simulink library "mach_lib"  (Simulink 6.3)
undefined symbols (not defined in the file): accel_cmd, aero_surf_qbar_off, aero_surf_qbar_on, altitude_stop, angular_rate_stop, att_cmd_select, att_trim_IC, att_type, att_type_numbers, bb_ellipsoid, bb_params, chi_trim_IC, command_time, compute_all_rate_cols, compute_all_vel_cols, constants, cosA, da_trim_IC, de_trim_IC, DiscIntNeverNeededParam, dr_trim_IC, dtsim, E_rwy, E_trim_IC, Ed_cmd, Ed_trim_IC, energy_stop, eow_boundary, full_surf_llim, full_surf_ulim, gain_var_struct, gam_cmd_descent, gam_cmd_preflare, gamdot_cmd_descent, gamdot_cmd_flare, gamdot_cmd_preflare, gamma_trim_IC, h_trim_IC, hd_cmd, hd_trim_IC, ideal_vel_Kb, integrate_start_time_sim, integrate_state_sim, llim, MACH, MACH_att_fb, MACH_gain_mat, MACH_mass_IC, MACH_pos_IC, MACH_pqr_Bmat_IC, MACH_pqr_IC, MACH_pqr_u_IC, MACH_quat_IC, MACH_throttle_IC, MACH_U_nom_IC, MACH_vel_Bmat_IC, MACH_vel_cvdnom_IC, MACH_vel_IC, MACH_vel_uold_IC, max_chi_cmd ... (+67)
libraries: simulink x75, mach_lib x27, utility_lib x25, model_lib x7, models x6
(part 1 of 6)
settings Model: Creator=spratt  LastModifiedBy=E700252  ExtModeAutoUpdateStatusClock=off  StrictBusMsg=None

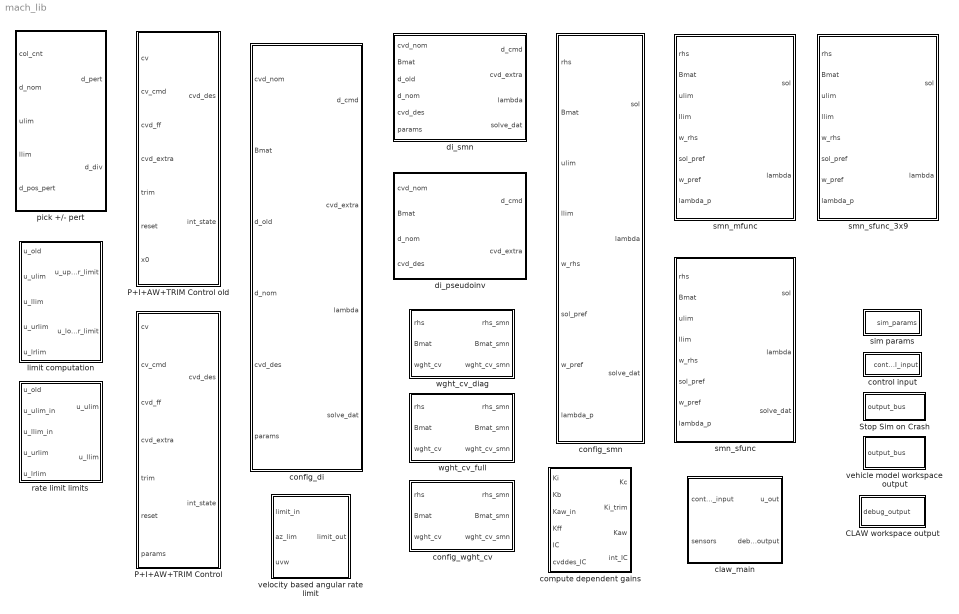
== system mach_lib ==
  CLAW workspace output : Subsystem
  P+I+AW+TRIM Control : Subsystem
  P+I+AW+TRIM Control old : Subsystem  mask{kb=MACH.xxx_Kb, ki=MACH.xxx_Ki, kc=MACH.xxx_Kc, kf=MACH.xxx_Kf, kaw=MACH.xxx_Kaw}
      mask prompts: kb "Kb (bandwidth gain)"; ki "Ki (integral gain)"; kc "Kc (command gain)"; kf "Kf (feedforward gain)"; kaw "Kaw (anti-windup gain)"
  Stop Sim on Crash : Subsystem
  claw_main : Subsystem  TreatAsAtomicUnit=on  SystemSampleTime=MACH.dt
  compute dependent gains : Subsystem
  config_di : Subsystem  BlockChoice=di_smn  mask{num_cv=0, num_u=0, wght_cv_type=0}
      settings: TemplateBlock=self  MemberBlocks=di_pseudoinv,di_smn
  config_smn : Subsystem  BlockChoice=smn_sfunc  mask{nr=num_cv, nc=num_u}
      settings: TemplateBlock=self  MemberBlocks=smn_mfunc,smn_sfunc,smn_sfunc_3x9
  config_wght_cv : Subsystem  BlockChoice=wght_cv_diag  mask{wght_cv_type=wght_cv_type}
      mask init:
      | try
      |     set_param(gcb, 'BlockChoice', wght_cv_type);
      | catch
      | %     disp(sprintf('resetting %s to default', gcb))
      | %     set_param(gcb, 'BlockChoice', 'wght_cv_diag');
      | end
      settings: TemplateBlock=self  MemberBlocks=wght_cv_diag,wght_cv_full
  control input : Subsystem  SystemSampleTime=MACH.dt
  di_pseudoinv : Subsystem
  di_smn : Subsystem
  limit computation : Subsystem
  pick +/- pert : Subsystem  mask{num_u=0}
  rate limit limits : Subsystem  mask{ulim=ulim, llim=llim}
      mask prompts: ulim "upper limit"; llim "lower limit"
  sim params : Subsystem
  smn_mfunc : Subsystem
  smn_sfunc : Subsystem  mask{sfunc_name=MACH.smn_sfunc_name}
      mask prompts: sfunc_name "S-function name"
      mask init:
      | block_name = [gcb '/S-Function'];
      | % disp(sprintf('S-Function name = %s',sfunc_name))
      | try
      |     set_param(block_name,'FunctionName',sfunc_name);
      | %     disp(sprintf('setting %s to %s',block_name,sfunc_name));
      | catch
      |     set_param(block_name,'FunctionName','smn_sfunc_3x9');
      | %     disp(sprintf('trouble setting smn_sfunc to %s, resetting %s to %s',sfunc_name,block_name,'smn_sfunc'));
      | end
  smn_sfunc_3x9 : Subsystem
  vehicle model workspace output : Subsystem
  velocity based angular rate limit : Subsystem  mask{q_idx=2}
      mask prompts: q_idx "q index"
  wght_cv_diag : Subsystem
  wght_cv_full : Subsystem

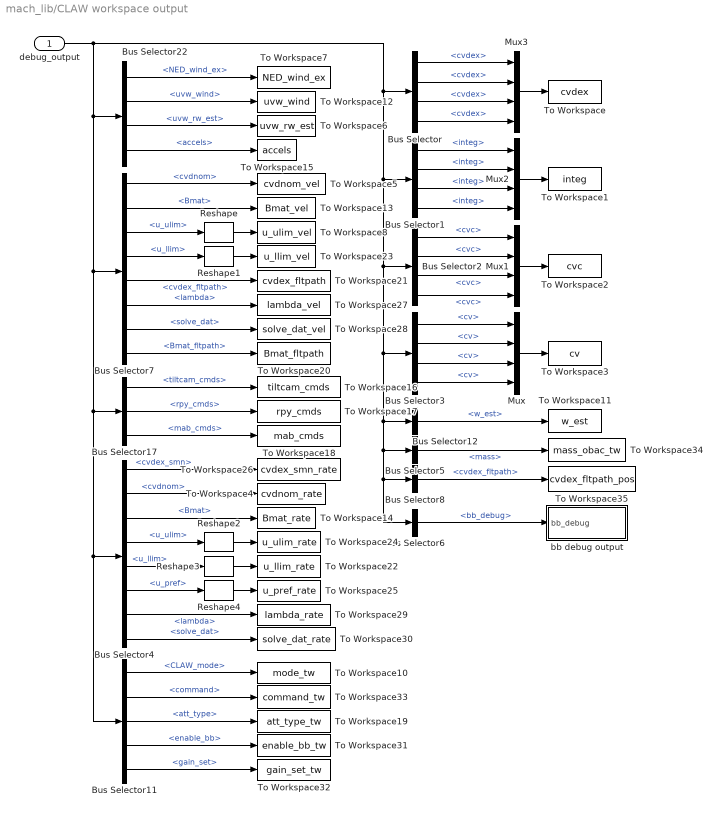
== system mach_lib/CLAW workspace output ==
  debug_output : Inport
  Bus Selector : BusSelector  OutputSignals=rate.cvdex,att.cvdex,vel.cvdex,pos.cvdex
  Bus Selector1 : BusSelector  OutputSignals=rate.integ,att.integ,vel.integ,pos.integ
  Bus Selector11 : BusSelector  OutputSignals=control_input.mode_sw.CLAW_mode,control_input.command,att_type,enable_bb,gain_set
  Bus Selector12 : BusSelector  OutputSignals=w_est_debug.w_est
  Bus Selector17 : BusSelector  OutputSignals=att.tiltcam_cmds,att.rpy_cmds,att.mab_cmds
  Bus Selector2 : BusSelector  OutputSignals=rate.cvc,att.cvc,vel.cvc,pos.cvc
  Bus Selector22 : BusSelector  OutputSignals=w_est_debug.NED_wind_ex,w_est_debug.uvw_wind,w_est_debug.uvw_rw_est,w_est_debug.accels
  Bus Selector3 : BusSelector  OutputSignals=rate.cv,att.cv,vel.cv,pos.cv
  Bus Selector4 : BusSelector  OutputSignals=rate.cvdex_smn,rate.cvdnom,rate.Bmat,rate.u_ulim,rate.u_llim,rate.u_pref,rate.lambda,rate.solve_dat
  Bus Selector5 : BusSelector  OutputSignals=mass
  Bus Selector6 : BusSelector  OutputSignals=rate.bb_debug
  Bus Selector7 : BusSelector  OutputSignals=vel.cvdnom,vel.Bmat,vel.u_ulim,vel.u_llim,vel.cvdex_fltpath,vel.lambda,vel.solve_dat,vel.Bmat_fltpath
  Bus Selector8 : BusSelector  OutputSignals=pos.cvdex_fltpath
  Mux{,1..3} (4 alike) : Mux
  Reshape{,1..4} (5 alike) : simulink/Math Operations/Reshape  OutputDimensionality=1-D array  OutputDimensions=[1,1]
  To Workspace : ToWorkspace  VariableName=cvdex  SampleTime=-1  SaveFormat=Array
  To Workspace1 : ToWorkspace  VariableName=integ  SampleTime=-1  SaveFormat=Array
  To Workspace10 : ToWorkspace  VariableName=mode_tw  SampleTime=-1  SaveFormat=Array
  To Workspace11 : ToWorkspace  VariableName=w_est  SampleTime=-1  SaveFormat=Array
  To Workspace12 : ToWorkspace  VariableName=uvw_wind  SampleTime=-1  SaveFormat=Array
  To Workspace13 : ToWorkspace  VariableName=Bmat_vel  SampleTime=-1  SaveFormat=Array
  To Workspace14 : ToWorkspace  VariableName=Bmat_rate  SampleTime=-1  SaveFormat=Array
  To Workspace15 : ToWorkspace  VariableName=accels  SampleTime=-1  SaveFormat=Array
  To Workspace16 : ToWorkspace  VariableName=tiltcam_cmds  SampleTime=-1  SaveFormat=Array
  To Workspace17 : ToWorkspace  VariableName=rpy_cmds  SampleTime=-1  SaveFormat=Array
  To Workspace18 : ToWorkspace  VariableName=mab_cmds  SampleTime=-1  SaveFormat=Array
  To Workspace19 : ToWorkspace  VariableName=att_type_tw  SampleTime=-1  SaveFormat=Array
  To Workspace2 : ToWorkspace  VariableName=cvc  SampleTime=-1  SaveFormat=Array
  To Workspace20 : ToWorkspace  VariableName=Bmat_fltpath  SampleTime=-1  SaveFormat=Array
  To Workspace21 : ToWorkspace  VariableName=cvdex_fltpath  SampleTime=-1  SaveFormat=Array
  To Workspace22 : ToWorkspace  VariableName=u_llim_rate  SampleTime=-1  SaveFormat=Array
  To Workspace23 : ToWorkspace  VariableName=u_llim_vel  SampleTime=-1  SaveFormat=Array
  To Workspace24 : ToWorkspace  VariableName=u_ulim_rate  SampleTime=-1  SaveFormat=Array
  To Workspace25 : ToWorkspace  VariableName=u_pref_rate  SampleTime=-1  SaveFormat=Array
  To Workspace26 : ToWorkspace  VariableName=cvdex_smn_rate  SampleTime=-1  SaveFormat=Array
  To Workspace27 : ToWorkspace  VariableName=lambda_vel  SampleTime=-1  SaveFormat=Array
  To Workspace28 : ToWorkspace  VariableName=solve_dat_vel  SampleTime=-1  SaveFormat=Array
  To Workspace29 : ToWorkspace  VariableName=lambda_rate  SampleTime=-1  SaveFormat=Array
  To Workspace3 : ToWorkspace  VariableName=cv  SampleTime=-1  SaveFormat=Array
  To Workspace30 : ToWorkspace  VariableName=solve_dat_rate  SampleTime=-1  SaveFormat=Array
  To Workspace31 : ToWorkspace  VariableName=enable_bb_tw  SampleTime=-1  SaveFormat=Array
  To Workspace32 : ToWorkspace  VariableName=gain_set_tw  SampleTime=-1  SaveFormat=Array
  To Workspace33 : ToWorkspace  VariableName=command_tw  SampleTime=-1  SaveFormat=Array
  To Workspace34 : ToWorkspace  VariableName=mass_obac_tw  SampleTime=-1  SaveFormat=Array
  To Workspace35 : ToWorkspace  VariableName=cvdex_fltpath_pos  SampleTime=-1  SaveFormat=Array
  To Workspace4 : ToWorkspace  VariableName=cvdnom_rate  SampleTime=-1  SaveFormat=Array
  To Workspace5 : ToWorkspace  VariableName=cvdnom_vel  SampleTime=-1  SaveFormat=Array
  To Workspace6 : ToWorkspace  VariableName=uvw_rw_est  SampleTime=-1  SaveFormat=Array
  To Workspace7 : ToWorkspace  VariableName=NED_wind_ex  SampleTime=-1  SaveFormat=Array
  To Workspace8 : ToWorkspace  VariableName=u_ulim_vel  SampleTime=-1  SaveFormat=Array
  bb debug output : Subsystem
  wires:
  Bus Selector8/1 -> To Workspace35/1  "<cvdex_fltpath>"
  Bus Selector6/1 -> bb debug output/1(bb_debug)  "<bb_debug>"
  Bus Selector5/1 -> To Workspace34/1  "<mass>"
  Bus Selector11/5 -> To Workspace32/1  "<gain_set>"
  Bus Selector11/4 -> To Workspace31/1  "<enable_bb>"
  Bus Selector7/8 -> To Workspace20/1  "<Bmat_fltpath>"
  Bus Selector4/8 -> To Workspace30/1  "<solve_dat>"
  Bus Selector4/7 -> To Workspace29/1  "<lambda>"
  Bus Selector7/7 -> To Workspace28/1  "<solve_dat>"
  Bus Selector7/6 -> To Workspace27/1  "<lambda>"
  Bus Selector4/1 -> To Workspace26/1  "<cvdex_smn>"
  Reshape4/1 -> To Workspace25/1
  Bus Selector4/6 -> Reshape4/1  "<u_pref>"
  Reshape3/1 -> To Workspace22/1
  Reshape2/1 -> To Workspace24/1
  Reshape1/1 -> To Workspace23/1
  Reshape/1 -> To Workspace8/1
  Bus Selector4/5 -> Reshape3/1  "<u_llim>"
  Bus Selector4/4 -> Reshape2/1  "<u_ulim>"
  Bus Selector4/3 -> To Workspace14/1  "<Bmat>"
  Bus Selector4/2 -> To Workspace4/1  "<cvdnom>"
  Bus Selector7/5 -> To Workspace21/1  "<cvdex_fltpath>"
  Bus Selector7/4 -> Reshape1/1  "<u_llim>"
  Bus Selector7/3 -> Reshape/1  "<u_ulim>"
  Bus Selector7/2 -> To Workspace13/1  "<Bmat>"
  Bus Selector7/1 -> To Workspace5/1  "<cvdnom>"
  Bus Selector22/4 -> To Workspace15/1  "<accels>"
  Bus Selector22/3 -> To Workspace6/1  "<uvw_rw_est>"
  Bus Selector22/2 -> To Workspace12/1  "<uvw_wind>"
  Bus Selector22/1 -> To Workspace7/1  "<NED_wind_ex>"
  Bus Selector11/2 -> To Workspace33/1  "<command>"
  Bus Selector11/1 -> To Workspace10/1  "<CLAW_mode>"
  Bus Selector17/3 -> To Workspace18/1  "<mab_cmds>"
  Bus Selector17/2 -> To Workspace17/1  "<rpy_cmds>"
  Bus Selector17/1 -> To Workspace16/1  "<tiltcam_cmds>"
  Bus Selector12/1 -> To Workspace11/1  "<w_est>"
  Bus Selector11/3 -> To Workspace19/1  "<att_type>"
  debug_output/1 -> Bus Selector4/1, Bus Selector11/1, Bus Selector17/1, Bus Selector7/1, Bus Selector22/1, Bus Selector8/1, Bus Selector6/1, Bus Selector5/1, Bus Selector12/1, Bus Selector3/1, Bus Selector2/1, Bus Selector1/1, Bus Selector/1
  Bus Selector3/1 -> Mux/1  "<cv>"
  Bus Selector3/2 -> Mux/2  "<cv>"
  Bus Selector3/3 -> Mux/3  "<cv>"
  Bus Selector3/4 -> Mux/4  "<cv>"
  Mux/1 -> To Workspace3/1
  Bus Selector2/1 -> Mux1/1  "<cvc>"
  Bus Selector2/2 -> Mux1/2  "<cvc>"
  Bus Selector2/3 -> Mux1/3  "<cvc>"
  Bus Selector2/4 -> Mux1/4  "<cvc>"
  Mux1/1 -> To Workspace2/1
  Bus Selector1/1 -> Mux2/1  "<integ>"
  Bus Selector1/2 -> Mux2/2  "<integ>"
  Bus Selector1/3 -> Mux2/3  "<integ>"
  Bus Selector1/4 -> Mux2/4  "<integ>"
  Mux2/1 -> To Workspace1/1
  Bus Selector/1 -> Mux3/1  "<cvdex>"
  Bus Selector/2 -> Mux3/2  "<cvdex>"
  Bus Selector/3 -> Mux3/3  "<cvdex>"
  Bus Selector/4 -> Mux3/4  "<cvdex>"
  Mux3/1 -> To Workspace/1

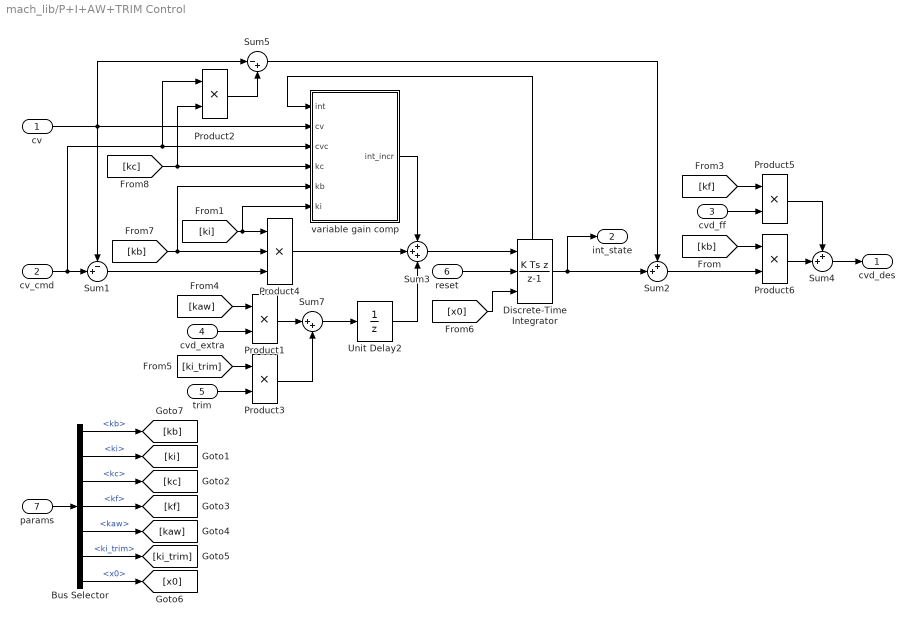
== system mach_lib/P+I+AW+TRIM Control ==
  cv : Inport
  cv_cmd : Inport  Port=2
  cvd_ff : Inport  Port=3
  cvd_extra : Inport  Port=4
  trim : Inport  Port=5
  reset : Inport  Port=6
  params : Inport  Port=7
  Bus Selector : BusSelector  OutputSignals=kb,ki,kc,kf,kaw,ki_trim,x0
  Discrete-Time Integrator : DiscreteIntegrator  IntegratorMethod=Integration: Backward Euler  ExternalReset=rising  InitialConditionSource=external  SampleTime=-1  ShowStatePort=on  ICPrevOutput=DiscIntNeverNeededParam  ICPrevScaledInput=DiscIntNeverNeededParam
  Product{1..3,5..6} (5 alike) : Product  RndMeth=Zero
  Product4 : Product  Inputs=3  RndMeth=Zero
  Sum1 : Sum  Inputs=-+|  SaturateOnIntegerOverflow=on  InputSameDT=on
  Sum2 : Sum  Inputs=++|  SaturateOnIntegerOverflow=on  InputSameDT=on
  Sum3 : Sum  Inputs=+++  SaturateOnIntegerOverflow=on  InputSameDT=on
  Sum4 : Sum  Inputs=++|  SaturateOnIntegerOverflow=on  InputSameDT=on
  Sum5 : Sum  Inputs=|-+  SaturateOnIntegerOverflow=on  InputSameDT=on
  Sum7 : Sum  Inputs=|++  SaturateOnIntegerOverflow=on  InputSameDT=on
  Unit Delay2 : UnitDelay  SampleTime=-1
  variable gain comp : Subsystem
  cvd_des : Outport
  int_state : Outport  Port=2
  wires:
  [x0] -> Discrete-Time Integrator/3
  Product5/1 -> Sum4/1
  Sum4/1 -> cvd_des/1
  Product6/1 -> Sum4/2
  trim/1 -> Product3/2
  Unit Delay2/1 -> Sum3/3
  Sum3/1 -> Discrete-Time Integrator/1
  Discrete-Time Integrator/1 -> int_state/1, Sum2/2
  cvd_extra/1 -> Product1/2
  reset/1 -> Discrete-Time Integrator/2
  Product3/1 -> Sum7/2
  Sum7/1 -> Unit Delay2/1
  Bus Selector/1 -> [kb]  "<kb>"
  Bus Selector/2 -> [ki]  "<ki>"
  Bus Selector/3 -> [kc]  "<kc>"
  Bus Selector/4 -> [kf]  "<kf>"
  Bus Selector/5 -> [kaw]  "<kaw>"
  Bus Selector/6 -> [ki_trim]  "<ki_trim>"
  [kaw] -> Product1/1
  Product1/1 -> Sum7/1
  [ki_trim] -> Product3/1
  Sum1/1 -> Product4/3
  [ki] -> Product4/1, variable gain comp/6(ki)
  [kb] -> Product6/1
  cvd_ff/1 -> Product5/2
  [kf] -> Product5/1
  params/1 -> Bus Selector/1
  Bus Selector/7 -> [x0]  "<x0>"
  cv/1 -> Sum1/1, Sum5/1, variable gain comp/2(cv)
  Sum2/1 -> Product6/2
  Product4/1 -> Sum3/2
  variable gain comp/1(int_incr) -> Sum3/1
  Discrete-Time Integrator/State -> variable gain comp/1(int)
  [kc] -> variable gain comp/4(kc), Product2/2
  Product2/1 -> Sum5/2
  Sum5/1 -> Sum2/1
  [kb] -> Product4/2, variable gain comp/5(kb)
  cv_cmd/1 -> variable gain comp/3(cvc), Product2/1, Sum1/2

== system mach_lib/P+I+AW+TRIM Control old ==
  cv : Inport
  cv_cmd : Inport  Port=2
  cvd_ff : Inport  Port=3
  cvd_extra : Inport  Port=4
  trim : Inport  Port=5
  reset : Inport  Port=6
  x0 : Inport  Port=7
  Discrete-Time Integrator : DiscreteIntegrator  IntegratorMethod=Integration: Backward Euler  ExternalReset=rising  InitialConditionSource=external  SampleTime=-1  ICPrevOutput=DiscIntNeverNeededParam  ICPrevScaledInput=DiscIntNeverNeededParam
  Kaw : Gain  Gain=kaw  SaturateOnIntegerOverflow=on
  Kb : Gain  Gain=kb  SaturateOnIntegerOverflow=on
  Kb1 : Gain  Gain=kb  SaturateOnIntegerOverflow=on
  Kc : Gain  Gain=kc  SaturateOnIntegerOverflow=on
  Kf : Gain  Gain=kf  SaturateOnIntegerOverflow=on
  Ki : Gain  Gain=ki  SaturateOnIntegerOverflow=on
  Sum1 : Sum  Inputs=|+-  SaturateOnIntegerOverflow=on  InputSameDT=on
  Sum2 : Sum  Inputs=|++  SaturateOnIntegerOverflow=on  InputSameDT=on
  Sum3 : Sum  Inputs=|++  SaturateOnIntegerOverflow=on  InputSameDT=on
  Sum4 : Sum  Inputs=++|  SaturateOnIntegerOverflow=on  InputSameDT=on
  Sum5 : Sum  Orientation=up  Inputs=++|  SaturateOnIntegerOverflow=on
  Sum6 : Sum  Inputs=-+|  SaturateOnIntegerOverflow=on  InputSameDT=on
  Unit Delay1 : UnitDelay  SampleTime=-1
  cvd_des : Outport
  int_state : Outport  Port=2
  wires:
  reset/1 -> Discrete-Time Integrator/2
  cvd_extra/1 -> Unit Delay1/1
  Discrete-Time Integrator/1 -> int_state/1, Sum2/1
  Sum3/1 -> Discrete-Time Integrator/1
  Ki/1 -> Sum3/1
  cv_cmd/1 -> Sum1/1, Kc/1
  Sum2/1 -> Kb/1
  cv/1 -> Sum1/2, Sum6/1
  Sum1/1 -> Kb1/1
  Kb1/1 -> Ki/1
  Sum5/1 -> Sum3/2
  Kaw/1 -> Sum5/1
  trim/1 -> Sum5/2
  Unit Delay1/1 -> Kaw/1
  Kb/1 -> Sum4/2
  Sum4/1 -> cvd_des/1
  cvd_ff/1 -> Kf/1
  Kf/1 -> Sum4/1
  Kc/1 -> Sum6/2
  Sum6/1 -> Sum2/2
  x0/1 -> Discrete-Time Integrator/3

== system mach_lib/Stop Sim on Crash ==
  note: If angular rates exceed 2 rad/sec, stop simulation
      |  because vehicle most likely crashed
  output_bus : Inport
  Abs : Abs  SaturateOnIntegerOverflow=on
  Bus Selector2 : BusSelector  OutputSignals=x,xdot
  Constant1 : Constant  Value=angular_rate_stop
  Constant2 : Constant  Value=altitude_stop
  Constant3 : Constant  Value=energy_stop
  MinMax : MinMax  Function=max  SaturateOnIntegerOverflow=on  InputSameDT=on
  NEh_dot : Selector  Elements=MACH.NEh_idx  InputPortWidth=trac_params.num_x
  Relational Operator1 : RelationalOperator  Operator=>
  Relational Operator2 : RelationalOperator  Operator=<
  Relational Operator3 : RelationalOperator  Operator=<
  Stop Simulation : Stop
  Stop Simulation1 : Stop
  Stop Simulation2 : Stop
  get specific energy : Subsystem
  h : Selector  Elements=MACH.NEh_idx(3)  InputPortWidth=MACH.num_x
  pqr : Selector  Elements=MACH.pqr_idx  InputPortWidth=trac_params.num_x
  wires:
  Abs/1 -> MinMax/1
  MinMax/1 -> Relational Operator1/1
  Relational Operator1/1 -> Stop Simulation/1
  Constant1/1 -> Relational Operator1/2
  pqr/1 -> Abs/1
  output_bus/1 -> Bus Selector2/1
  Constant2/1 -> Relational Operator2/2
  h/1 -> get specific energy/1(h), Relational Operator2/1
  Relational Operator2/1 -> Stop Simulation1/1
  Constant3/1 -> Relational Operator3/2
  get specific energy/1(energy) -> Relational Operator3/1
  Relational Operator3/1 -> Stop Simulation2/1
  Bus Selector2/1 -> h/1, pqr/1  "<x>"
  NEh_dot/1 -> get specific energy/2(NEh_dot)
  Bus Selector2/2 -> NEh_dot/1  "<xdot>"

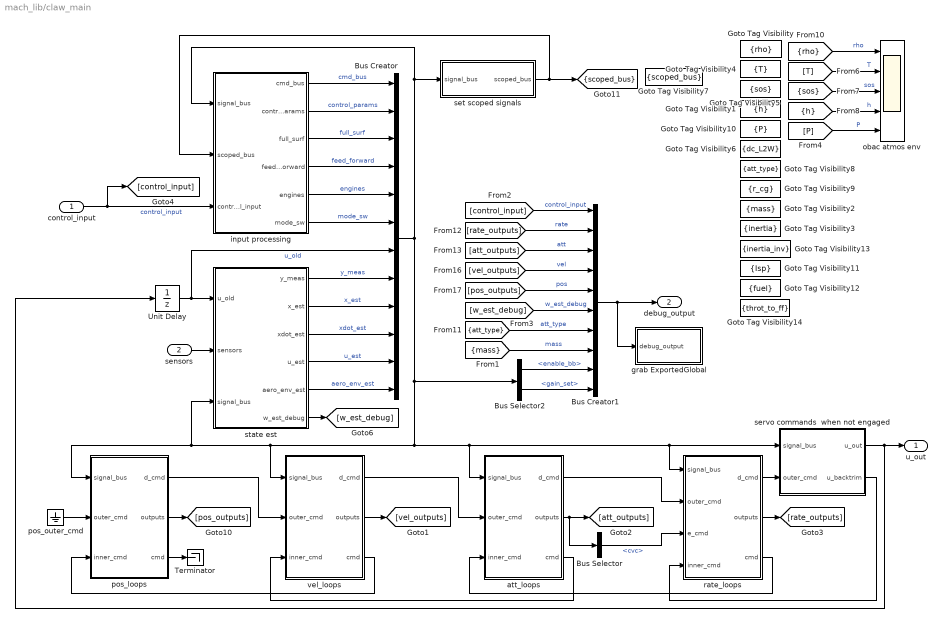
== system mach_lib/claw_main ==
  control_input : Inport
      settings: BusObject=control_input_bus
  sensors : Inport  Port=2
  Bus Creator : BusCreator  Inputs=12
  Bus Creator1 : BusCreator  Inputs=10
      settings: BusObject=CLAW_DEBUG_OUTPUT_BUS
  Bus Selector : BusSelector  OutputSignals=cvc
  Bus Selector2 : BusSelector  OutputSignals=control_params.enable_bb,control_params.gain_set
  Goto Tag Visibility : GotoTagVisibility  GotoTag=rho
  Goto Tag Visibility1 : GotoTagVisibility  GotoTag=h
  Goto Tag Visibility10 : GotoTagVisibility  GotoTag=P
  Goto Tag Visibility11 : GotoTagVisibility  GotoTag=Isp
  Goto Tag Visibility12 : GotoTagVisibility  GotoTag=fuel
  Goto Tag Visibility13 : GotoTagVisibility  GotoTag=inertia_inv
  Goto Tag Visibility14 : GotoTagVisibility  GotoTag=throt_to_ff
  Goto Tag Visibility2 : GotoTagVisibility  GotoTag=mass
  Goto Tag Visibility3 : GotoTagVisibility  GotoTag=inertia
  Goto Tag Visibility4 : GotoTagVisibility  GotoTag=T
  Goto Tag Visibility5 : GotoTagVisibility  GotoTag=sos
  Goto Tag Visibility6 : GotoTagVisibility  GotoTag=dc_L2W
  Goto Tag Visibility7 : GotoTagVisibility  GotoTag=scoped_bus
  Goto Tag Visibility8 : GotoTagVisibility  GotoTag=att_type
  Goto Tag Visibility9 : GotoTagVisibility  GotoTag=r_cg
  Terminator : Terminator
  Unit Delay : UnitDelay  X0=MACH_U_nom_IC  SampleTime=-1
  att_loops : Subsystem
  grab ExportedGlobal : Subsystem
  input processing : Subsystem
  obac atmos env : Scope  NumInputPorts=5
      settings: YMin=-5~-5~-5~-5~-5  YMax=5~5~5~5~5  SaveName=ScopeData2
  pos_loops : Subsystem
      settings: RTWSystemCode=Function
  pos_outer_cmd : Ground
  rate_loops : Subsystem
      settings: RTWSystemCode=Function
  servo commands  when not engaged : Subsystem
  set scoped signals : Subsystem
  state est : Subsystem
  vel_loops : Subsystem
      settings: RTWSystemCode=Function
  u_out : Outport
  debug_output : Outport  Port=2
  tag scope: scoped_bus=scoped
  wires:
  Bus Selector/1 -> rate_loops/3(e_cmd)  "<cvc>"
  [control_input] -> Bus Creator1/1  "control_input"
  input processing/1(cmd_bus) -> Bus Creator/1  "cmd_bus"
  control_input/1 -> [control_input], input processing/3(control_input)  "control_input"
  Bus Selector2/2 -> Bus Creator1/10  "<gain_set>"
  Bus Selector2/1 -> Bus Creator1/9  "<enable_bb>"
  [mass] -> Bus Creator1/8  "mass"
  set scoped signals/1(scoped_bus) -> input processing/2(scoped_bus), [scoped_bus]
  input processing/4(feed_forward) -> Bus Creator/4  "feed_forward"
  input processing/3(full_surf) -> Bus Creator/3  "full_surf"
  state est/5(aero_env_est) -> Bus Creator/12  "aero_env_est"
  [P] -> obac atmos env/5  "P"
  [rho] -> obac atmos env/1  "rho"
  [T] -> obac atmos env/2  "T"
  [sos] -> obac atmos env/3  "sos"
  [h] -> obac atmos env/4  "h"
  input processing/2(control_params) -> Bus Creator/2  "control_params"
  [att_type] -> Bus Creator1/7  "att_type"
  [w_est_debug] -> Bus Creator1/6  "w_est_debug"
  state est/6(w_est_debug) -> [w_est_debug]
  pos_outer_cmd/1 -> pos_loops/2(outer_cmd)
  servo commands  when not engaged/1(u_out) -> Unit Delay/1, u_out/1
  state est/1(y_meas) -> Bus Creator/8  "y_meas"
  state est/2(x_est) -> Bus Creator/9  "x_est"
  state est/3(xdot_est) -> Bus Creator/10  "xdot_est"
  state est/4(u_est) -> Bus Creator/11  "u_est"
  servo commands  when not engaged/2(u_backtrim) -> rate_loops/4(inner_cmd)
  vel_loops/3(cmd) -> pos_loops/3(inner_cmd)
  sensors/1 -> state est/2(sensors)
  Unit Delay/1 -> Bus Creator/7, state est/1(u_old)  "u_old"
  Bus Creator1/1 -> grab ExportedGlobal/1(debug_output), debug_output/1
  rate_loops/2(outputs) -> [rate_outputs]
  att_loops/2(outputs) -> Bus Selector/1, [att_outputs]
  vel_loops/2(outputs) -> [vel_outputs]
  pos_loops/1(d_cmd) -> vel_loops/2(outer_cmd)
  rate_loops/3(cmd) -> att_loops/3(inner_cmd)
  att_loops/3(cmd) -> vel_loops/3(inner_cmd)
  pos_loops/3(cmd) -> Terminator/1
  Bus Creator/1 -> set scoped signals/1(signal_bus), input processing/1(signal_bus), Bus Selector2/1, state est/3(signal_bus), pos_loops/1(signal_bus), vel_loops/1(signal_bus), servo commands  when not engaged/1(signal_bus), rate_loops/1(signal_bus), att_loops/1(signal_bus)
  rate_loops/1(d_cmd) -> servo commands  when not engaged/2(outer_cmd)
  vel_loops/1(d_cmd) -> att_loops/2(outer_cmd)
  att_loops/1(d_cmd) -> rate_loops/2(outer_cmd)
  [rate_outputs] -> Bus Creator1/2  "rate"
  [att_outputs] -> Bus Creator1/3  "att"
  [vel_outputs] -> Bus Creator1/4  "vel"
  [pos_outputs] -> Bus Creator1/5  "pos"
  pos_loops/2(outputs) -> [pos_outputs]
  input processing/5(engines) -> Bus Creator/5  "engines"
  input processing/6(mode_sw) -> Bus Creator/6  "mode_sw"

== system mach_lib/compute dependent gains ==
  Ki : Inport
  Kb : Inport  Port=2
  Kaw_in : Inport  Port=3
  Kff : Inport  Port=4
  IC : Inport  Port=5
  cvddes_IC : Inport  Port=6
  Compare To Zero : simulink/Logic and Bit Operations/Compare To Zero  relop=>  LogicOutDataTypeMode=boolean  ZeroCross=off
  Constant : Constant
  Constant1 : Constant  Value=MACH.trim_loop_gain
  Constant2 : Constant
  Constant3 : Constant
  Constant4 : Constant  Value=0
  Divide : Product  Inputs=//**  OutScaling=2^-10
  Divide1 : Product  Inputs=**  OutScaling=2^-10
  Divide2 : Product  Inputs=**  OutScaling=2^-10
  Divide3 : Product  Inputs=/*  OutScaling=2^-10
  Gain : Gain  Gain=4
  Gain1 : Gain  Gain=0.5
  Math Function : Math  Operator=sqrt  SaturateOnIntegerOverflow=on
  Math Function1 : Math  Operator=sqrt  SaturateOnIntegerOverflow=on
  Sum : Sum  Inputs=|-+
  Sum1 : Sum  Inputs=|++
  Sum2 : Sum  Inputs=-+|
  Sum3 : Sum  Inputs=|++
  Switch : Switch  Threshold=0.25
  Switch1 : Switch  Threshold=1
  Switch2 : Switch  Threshold=1
  Kc : Outport
  Ki_trim : Outport  Port=2
  Kaw : Outport  Port=3
  int_IC : Outport  Port=4
  wires:
  Sum1/1 -> Gain1/1
  Math Function1/1 -> Sum1/1
  Sum/1 -> Math Function1/1
  Constant/1 -> Sum1/2, Sum/2
  Gain/1 -> Sum/1
  Math Function/1 -> Switch/1
  Gain1/1 -> Switch/3
  Ki/1 -> Switch/2, Math Function/1, Gain/1, Compare To Zero/1
  Switch/1 -> Switch1/3, Divide/2
  Constant1/1 -> Divide/3
  Divide/1 -> Ki_trim/1
  Compare To Zero/1 -> Divide/4, Divide1/1
  Kaw_in/1 -> Divide1/2
  Divide1/1 -> Kaw/1
  Constant2/1 -> Sum2/2
  Sum2/1 -> Divide2/1
  IC/1 -> Divide2/2
  Constant3/1 -> Switch1/1
  Kff/1 -> Switch1/2, Switch2/2
  Switch1/1 -> Sum2/1, Kc/1
  Divide3/1 -> Sum3/2
  Divide2/1 -> Sum3/1
  cvddes_IC/1 -> Divide3/2
  Kb/1 -> Divide/1, Divide3/1
  Constant4/1 -> Switch2/1
  Switch2/1 -> int_IC/1
  Sum3/1 -> Switch2/3

== system mach_lib/config_di ==
  cvd_nom : Inport
  Bmat : Inport  Port=2
  d_old : Inport  Port=3
  d_nom : Inport  Port=4
  cvd_des : Inport  Port=5
  params : Inport  Port=6
  di_smn : mach_lib/di_smn
  d_cmd : Outport
  cvd_extra : Outport  Port=2
  lambda : Outport  Port=3
  solve_dat : Outport  Port=4
  wires:
  cvd_nom/1 -> di_smn/1
  Bmat/1 -> di_smn/2
  d_old/1 -> di_smn/3
  d_nom/1 -> di_smn/4
  cvd_des/1 -> di_smn/5
  params/1 -> di_smn/6
  di_smn/1 -> d_cmd/1
  di_smn/2 -> cvd_extra/1
  di_smn/3 -> lambda/1
  di_smn/4 -> solve_dat/1

== system mach_lib/config_smn ==
  rhs : Inport
  Bmat : Inport  Port=2
  ulim : Inport  Port=3
  llim : Inport  Port=4
  w_rhs : Inport  Port=5
  sol_pref : Inport  Port=6
  w_pref : Inport  Port=7
  lambda_p : Inport  Port=8
  smn_sfunc : mach_lib/smn_sfunc  sfunc_name=smn_sfunc_name
  sol : Outport
  lambda : Outport  Port=2
  solve_dat : Outport  Port=3
  wires:
  rhs/1 -> smn_sfunc/1
  Bmat/1 -> smn_sfunc/2
  ulim/1 -> smn_sfunc/3
  llim/1 -> smn_sfunc/4
  w_rhs/1 -> smn_sfunc/5
  sol_pref/1 -> smn_sfunc/6
  w_pref/1 -> smn_sfunc/7
  lambda_p/1 -> smn_sfunc/8
  smn_sfunc/1 -> sol/1
  smn_sfunc/2 -> lambda/1
  smn_sfunc/3 -> solve_dat/1

== system mach_lib/config_wght_cv ==
  rhs : Inport
  Bmat : Inport  Port=2
  wght_cv : Inport  Port=3
  wght_cv_diag : mach_lib/wght_cv_diag
  rhs_smn : Outport
  Bmat_smn : Outport  Port=2
  wght_cv_smn : Outport  Port=3
  wires:
  rhs/1 -> wght_cv_diag/1
  Bmat/1 -> wght_cv_diag/2
  wght_cv/1 -> wght_cv_diag/3
  wght_cv_diag/1 -> rhs_smn/1
  wght_cv_diag/2 -> Bmat_smn/1
  wght_cv_diag/3 -> wght_cv_smn/1

== system mach_lib/control input ==
  Rate Transition1 : RateTransition  OutPortSampleTime=MACH.dt
  form control input : Subsystem  SystemSampleTime=MACH.dt
  generate commands : Subsystem
  ideal responses : model_lib/ideal responses
  control_input : Outport
  wires:
  generate commands/1(cmd_bus) -> form control input/1(cmd_bus)
  form control input/1(control_input) -> Rate Transition1/1
  Rate Transition1/1 -> control_input/1, ideal responses/1

== system mach_lib/di_pseudoinv ==
  cvd_nom : Inport
  Bmat : Inport  Port=2
  d_nom : Inport  Port=3
  cvd_des : Inport  Port=4
  Product : Product  Multiplication=Matrix(*)  SaturateOnIntegerOverflow=on  InputSameDT=on
  Sum : Sum  Inputs=|+-  SaturateOnIntegerOverflow=on  InputSameDT=on
  Sum4 : Sum  Inputs=|++  SaturateOnIntegerOverflow=on  InputSameDT=on
  Sum5 : Sum  Inputs=+-|  SaturateOnIntegerOverflow=on  InputSameDT=on
  pseudoinv : Subsystem
  d_cmd : Outport
  cvd_extra : Outport  Port=2
  wires:
  Product/1 -> Sum5/1
  cvd_des/1 -> Sum/1
  cvd_nom/1 -> Sum/2
  Bmat/1 -> pseudoinv/2(Bmat), Product/1
  Sum/1 -> pseudoinv/1(rhs), Sum5/2
  pseudoinv/1(sol) -> Sum4/1, Product/2
  d_nom/1 -> Sum4/2
  Sum4/1 -> d_cmd/1
  Sum5/1 -> cvd_extra/1

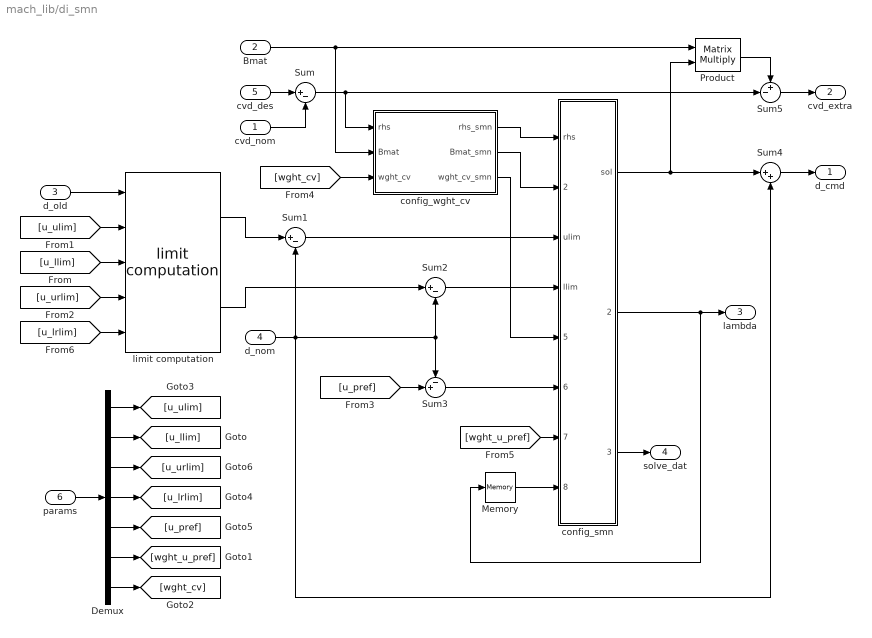
== system mach_lib/di_smn ==
  cvd_nom : Inport
  Bmat : Inport  Port=2
  d_old : Inport  Port=3
  d_nom : Inport  Port=4
  cvd_des : Inport  Port=5
  params : Inport  Port=6
  Demux : Demux  Outputs=7  BusSelectionMode=on
  Memory : Memory  InheritSampleTime=on
  Product : Product  Multiplication=Matrix(*)  SaturateOnIntegerOverflow=on  InputSameDT=on
  Sum : Sum  Inputs=|+-  SaturateOnIntegerOverflow=on  InputSameDT=on
  Sum1 : Sum  Inputs=|+-  SaturateOnIntegerOverflow=on  InputSameDT=on
  Sum2 : Sum  Inputs=|+-  SaturateOnIntegerOverflow=on  InputSameDT=on
  Sum3 : Sum  Inputs=-+|  SaturateOnIntegerOverflow=on  InputSameDT=on
  Sum4 : Sum  Inputs=|++  SaturateOnIntegerOverflow=on  InputSameDT=on
  Sum5 : Sum  Inputs=+-|  SaturateOnIntegerOverflow=on  InputSameDT=on
  config_smn : Subsystem  BlockChoice=smn_sfunc  mask{nr=num_cv, nc=num_u}
      link override smn_mfile: nr=num_cv  nc=num_u
      link override smn_sfunc: nr=num_cv  nc=num_u
      settings: AttributesFormatString=%<BlockChoice>  TemplateBlock=mach_lib/config_smn  MemberBlocks=smn_mfunc,smn_sfunc,smn_sfunc_3x9,smn_sfunc_old
  config_wght_cv : Subsystem  BlockChoice=wght_cv_diag  mask{wght_cv_type=wght_cv_type}
      mask init:
      | try
      |     set_param(gcb, 'BlockChoice', wght_cv_type);
      | catch
      |     disp(sprintf('resetting %s to default', gcb))
      |     set_param(gcb, 'BlockChoice', 'wght_cv_diag');
      | end
      settings: AttributesFormatString=%<BlockChoice>  TemplateBlock=mach_lib/config_wght_cv  MemberBlocks=wght_cv_diag,wght_cv_full
  limit computation : mach_lib/limit computation
  d_cmd : Outport
  cvd_extra : Outport  Port=2
  lambda : Outport  Port=3
  solve_dat : Outport  Port=4
  wires:
  [u_ulim] -> limit computation/2
  [u_llim] -> limit computation/3
  [u_urlim] -> limit computation/4
  d_old/1 -> limit computation/1
  Demux/7 -> [wght_cv]
  Demux/6 -> [wght_u_pref]
  Demux/5 -> [u_pref]
  Demux/4 -> [u_lrlim]
  Demux/2 -> [u_llim]
  Demux/1 -> [u_ulim]
  params/1 -> Demux/1
  [wght_u_pref] -> config_smn/7(w_pref)
  config_wght_cv/3(wght_cv_smn) -> config_smn/5(w_rhs)
  [u_pref] -> Sum3/2
  Product/1 -> Sum5/1
  cvd_des/1 -> Sum/1
  cvd_nom/1 -> Sum/2
  Bmat/1 -> Product/1, config_wght_cv/2(Bmat)
  Sum/1 -> Sum5/2, config_wght_cv/1(rhs)
  config_smn/1(sol) -> Sum4/1, Product/2
  limit computation/1 -> Sum1/1
  limit computation/2 -> Sum2/1
  d_nom/1 -> Sum4/2, Sum3/1, Sum2/2, Sum1/2
  Sum3/1 -> config_smn/6(sol_pref)
  Sum2/1 -> config_smn/4(llim)
  Sum1/1 -> config_smn/3(ulim)
  config_smn/2(lambda) -> Memory/1, lambda/1
  Memory/1 -> config_smn/8(lambda_p)
  Sum4/1 -> d_cmd/1
  Sum5/1 -> cvd_extra/1
  config_wght_cv/1(rhs_smn) -> config_smn/1(rhs)
  config_wght_cv/2(Bmat_smn) -> config_smn/2(Bmat)
  [wght_cv] -> config_wght_cv/3(wght_cv)
  [u_lrlim] -> limit computation/5
  Demux/3 -> [u_urlim]
  config_smn/3(solve_dat) -> solve_dat/1

== system mach_lib/limit computation ==
  u_old : Inport
  u_ulim : Inport  Port=2
  u_llim : Inport  Port=3
  u_urlim : Inport  Port=4
  u_lrlim : Inport  Port=5
  Gain : Gain  Gain=MACH.dt  SaturateOnIntegerOverflow=on
  Gain1 : Gain  Gain=MACH.dt  SaturateOnIntegerOverflow=on
  MinMax : MinMax  Inputs=2  SaturateOnIntegerOverflow=on  InputSameDT=on
  MinMax1 : MinMax  Function=max  Inputs=2  SaturateOnIntegerOverflow=on  InputSameDT=on
  MinMax2 : MinMax  Function=max  Inputs=2  SaturateOnIntegerOverflow=on  InputSameDT=on
  MinMax3 : MinMax  Inputs=2  SaturateOnIntegerOverflow=on  InputSameDT=on
  Sum1 : Sum  SaturateOnIntegerOverflow=on  InputSameDT=on
  Sum2 : Sum  SaturateOnIntegerOverflow=on  InputSameDT=on
  u_upper_limit : Outport
  u_lower_limit : Outport  Port=2
  wires:
  Gain/1 -> Sum1/2
  u_old/1 -> Sum1/1, Sum2/1
  MinMax1/1 -> MinMax/1
  u_llim/1 -> MinMax1/2, MinMax2/2
  u_ulim/1 -> MinMax/2, MinMax3/2
  u_urlim/1 -> Gain/1
  Sum2/1 -> MinMax1/1
  MinMax3/1 -> MinMax2/1
  Sum1/1 -> MinMax3/1
  MinMax/1 -> u_lower_limit/1
  MinMax2/1 -> u_upper_limit/1
  u_lrlim/1 -> Gain1/1
  Gain1/1 -> Sum2/2

== system mach_lib/pick +/- pert ==
  note: Original modified to always allow
      | negative delta if positive fails
  col_cnt : Inport
  d_nom : Inport  Port=2
  ulim : Inport  Port=3
  llim : Inport  Port=4
  d_pos_pert : Inport  Port=5
  Relational Operator : RelationalOperator  Operator=<=  InputSameDT=on
  Reshape : simulink/Math Operations/Reshape  OutputDimensionality=1-D array  OutputDimensions=[1,1]
  Selector : Selector  ElementSrc=External  Elements=[3]  ColumnSrc=External  InputPortWidth=num_u
  Selector1 : Selector  ElementSrc=External  Elements=[3]  ColumnSrc=External  InputPortWidth=num_u
  Selector4 : Selector  ElementSrc=External  Elements=[3]  ColumnSrc=External  InputPortWidth=num_u
  Selector5 : Selector  InputType=Matrix  ElementSrc=External  Elements=[3]  Rows=-1  ColumnSrc=External  InputPortWidth=MACH.vel_num_u
  Sum1 : Sum  Inputs=+|-  SaturateOnIntegerOverflow=on  InputSameDT=on
  Sum2 : Sum  Inputs=-+|  SaturateOnIntegerOverflow=on  InputSameDT=on
  Sum3 : Sum  Inputs=|++  SaturateOnIntegerOverflow=on  InputSameDT=on
  Switch : Switch  Threshold=0.5  SaturateOnIntegerOverflow=on  InputSameDT=on
  Terminator : Terminator
  d_pert : Outport
  d_div : Outport  Port=2
  wires:
  d_pos_pert/1 -> Selector5/1
  [cc] -> Selector5/2
  Selector5/1 -> Reshape/1
  Selector1/1 -> Relational Operator/2
  Selector/1 -> Relational Operator/1
  [cc] -> Selector4/2
  [cc] -> Selector/2
  [cc] -> Selector1/2
  col_cnt/1 -> [cc]
  Sum1/1 -> Selector4/1
  Selector4/1 -> d_div/1
  Switch/1 -> Sum1/1, d_pert/1
  Relational Operator/1 -> Switch/2
  Sum2/1 -> Switch/3  "d-"
  Sum3/1 -> Switch/1, Selector/1  "d+"
  d_nom/1 -> Sum3/1, Sum2/2, Sum1/2
  Reshape/1 -> Sum2/1, Sum3/2
  ulim/1 -> Selector1/1
  llim/1 -> Terminator/1

== system mach_lib/rate limit limits ==
  u_old : Inport
  u_ulim_in : Inport  Port=2
  u_llim_in : Inport  Port=3
  u_urlim : Inport  Port=4
  u_lrlim : Inport  Port=5
  Constant1 : Constant  Value=llim
  Constant3 : Constant  Value=ulim
  Gain : Gain  Gain=MACH.dt  SaturateOnIntegerOverflow=on
  Gain1 : Gain  Gain=MACH.dt  SaturateOnIntegerOverflow=on
  MinMax1 : MinMax  Function=max  Inputs=2
  MinMax2 : MinMax  Inputs=2
  MinMax3 : MinMax  Function=max  Inputs=2  SaturateOnIntegerOverflow=on  InputSameDT=on
  MinMax4 : MinMax  Inputs=2  SaturateOnIntegerOverflow=on  InputSameDT=on
  Sum1 : Sum  SaturateOnIntegerOverflow=on  InputSameDT=on
  Sum2 : Sum  SaturateOnIntegerOverflow=on  InputSameDT=on
  u_ulim : Outport
  u_llim : Outport  Port=2
  wires:
  MinMax4/1 -> u_llim/1
  MinMax3/1 -> u_ulim/1
  MinMax1/1 -> MinMax4/2
  u_urlim/1 -> Gain/1
  Sum1/1 -> MinMax4/1
  MinMax2/1 -> MinMax3/1
  Sum2/1 -> MinMax3/2
  Gain/1 -> Sum1/2
  u_old/1 -> Sum1/1, Sum2/2
  Constant1/1 -> MinMax1/1
  u_llim_in/1 -> MinMax1/2
  Constant3/1 -> MinMax2/1
  u_ulim_in/1 -> MinMax2/2
  u_lrlim/1 -> Gain1/1
  Gain1/1 -> Sum2/1

== system mach_lib/sim params ==
  Bus Creator : BusCreator  Inputs=5
  From Workspace2 : FromWorkspace  VariableName=use_held_aero_trac_fw  SampleTime=dtsim  Interpolate=off  OutputAfterFinalValue=Holding final value
  Rate Transition : RateTransition  OutPortSampleTime=dtsim
  Step : Step  Time=integrate_start_time_sim  After=integrate_state_sim  SampleTime=dtsim
  effector limits : Subsystem
  engines : Subsystem
  winds : Subsystem
  sim_params : Outport
  wires:
  From Workspace2/1 -> Bus Creator/5  "use_held_aero_trac_sw"
  engines/1(engines) -> Bus Creator/4  "engines"
  Bus Creator/1 -> Rate Transition/1
  effector limits/1(effector_limits) -> Bus Creator/2  "effector_limits"
  winds/1(winds) -> Bus Creator/3  "NED_wind"
  Step/1 -> Bus Creator/1  "integrate_state_sw"
  Rate Transition/1 -> sim_params/1

== system mach_lib/smn_mfunc ==
  rhs : Inport
  Bmat : Inport  Port=2
  ulim : Inport  Port=3
  llim : Inport  Port=4
  w_rhs : Inport  Port=5
  sol_pref : Inport  Port=6
  w_pref : Inport  Port=7
  lambda_p : Inport  Port=8
  Demux : Demux  Outputs=[nc 1]
  MATLAB Fcn : MATLABFcn  MATLABFcn=smn_mfunc(u)  OutputDimensions=nc+1
  Mux : Mux  Inputs=10
  Reshape : simulink/Math Operations/Reshape  OutputDimensionality=1-D array  OutputDimensions=[1,1]
  ncolumns : Constant  Value=nc
  nrows : Constant  Value=nr
  sol : Outport
  lambda : Outport  Port=2
  wires:
  Demux/2 -> lambda/1
  Reshape/1 -> Mux/3
  ncolumns/1 -> Mux/2
  nrows/1 -> Mux/1
  Demux/1 -> sol/1
  MATLAB Fcn/1 -> Demux/1
  Mux/1 -> MATLAB Fcn/1
  Bmat/1 -> Reshape/1
  rhs/1 -> Mux/4
  llim/1 -> Mux/5
  lambda_p/1 -> Mux/10
  w_pref/1 -> Mux/9
  sol_pref/1 -> Mux/8
  w_rhs/1 -> Mux/7
  ulim/1 -> Mux/6

== system mach_lib/smn_sfunc ==
  rhs : Inport
  Bmat : Inport  Port=2
  ulim : Inport  Port=3
  llim : Inport  Port=4
  w_rhs : Inport  Port=5
  sol_pref : Inport  Port=6
  w_pref : Inport  Port=7
  lambda_p : Inport  Port=8
  Mux : Mux  Inputs=10
  Reshape : simulink/Math Operations/Reshape  OutputDimensionality=1-D array  OutputDimensions=[1,1]
  Reshape1 : simulink/Math Operations/Reshape  OutputDimensionality=Customize  OutputDimensions=[22 nc]
  S-Function : S-Function  FunctionName=smn_sfunc_gam_mpass_epsposdef
  Selector : Selector  Elements=1:nc  InputPortWidth=smn_sfunc_output_dim
  Selector1 : Selector  Elements=nc+1  InputPortWidth=smn_sfunc_output_dim
  Selector2 : Selector  Elements=[1:22*nc] + nc + 1  InputPortWidth=smn_sfunc_output_dim
  ncolumns : Constant  Value=nc
  nrows : Constant  Value=nr
  sol : Outport
  lambda : Outport  Port=2
  solve_dat : Outport  Port=3
  wires:
  Selector1/1 -> lambda/1
  Reshape/1 -> Mux/3
  ncolumns/1 -> Mux/2
  nrows/1 -> Mux/1
  S-Function/1 -> Selector/1, Selector1/1, Selector2/1
  Mux/1 -> S-Function/1
  Bmat/1 -> Reshape/1
  rhs/1 -> Mux/4
  llim/1 -> Mux/5
  lambda_p/1 -> Mux/10
  w_pref/1 -> Mux/9
  sol_pref/1 -> Mux/8
  w_rhs/1 -> Mux/7
  ulim/1 -> Mux/6
  Selector/1 -> sol/1
  Selector2/1 -> Reshape1/1
  Reshape1/1 -> solve_dat/1

== system mach_lib/smn_sfunc_3x9 ==
  rhs : Inport
  Bmat : Inport  Port=2
  ulim : Inport  Port=3
  llim : Inport  Port=4
  w_rhs : Inport  Port=5
  sol_pref : Inport  Port=6
  w_pref : Inport  Port=7
  lambda_p : Inport  Port=8
  Mux : Mux  Inputs=10
  Reshape : simulink/Math Operations/Reshape  OutputDimensionality=1-D array  OutputDimensions=[1,1]
  S-Function : S-Function  FunctionName=smn_sfunc_3x9  SFunctionModules=smn_sfunc_wrapper
  Selector : Selector  Elements=1:nc  InputPortWidth=10
  Selector1 : Selector  Elements=nc+1  InputPortWidth=10
  ncolumns : Constant  Value=nc
  nrows : Constant  Value=nr
  sol : Outport
  lambda : Outport  Port=2
  wires:
  Selector/1 -> sol/1
  ulim/1 -> Mux/6
  w_rhs/1 -> Mux/7
  sol_pref/1 -> Mux/8
  w_pref/1 -> Mux/9
  lambda_p/1 -> Mux/10
  llim/1 -> Mux/5
  rhs/1 -> Mux/4
  Bmat/1 -> Reshape/1
  Mux/1 -> S-Function/1
  S-Function/1 -> Selector1/1, Selector/1
  nrows/1 -> Mux/1
  ncolumns/1 -> Mux/2
  Reshape/1 -> Mux/3
  Selector1/1 -> lambda/1

== system mach_lib/vehicle model workspace output ==
  output_bus : Inport
  Bus Selector2 : BusSelector  OutputSignals=u_servo,x,xdot,NED_wind,y_mkplt,u_cmd,u_ulim,u_llim
  To Workspace : ToWorkspace  VariableName=x  SampleTime=dtsim  SaveFormat=Array
  To Workspace1 : ToWorkspace  VariableName=u_cmd  SampleTime=MACH.dt  SaveFormat=Array
  To Workspace12 : ToWorkspace  VariableName=winds  SampleTime=dtsim  SaveFormat=Array
  To Workspace2 : ToWorkspace  VariableName=full_surf_trac_llim  SampleTime=MACH.dt  SaveFormat=Array
  To Workspace3 : ToWorkspace  VariableName=full_surf_trac_ulim  SampleTime=MACH.dt  SaveFormat=Array
  To Workspace5 : ToWorkspace  VariableName=xdot  SampleTime=dtsim  SaveFormat=Array
  To Workspace6 : ToWorkspace  VariableName=u_servo  SampleTime=MACH.dt  SaveFormat=Array
  To Workspace7 : ToWorkspace  VariableName=y  SampleTime=dtsim  SaveFormat=Array
  wires:
  Bus Selector2/1 -> To Workspace6/1  "<u_servo>"
  Bus Selector2/2 -> To Workspace/1  "<x>"
  Bus Selector2/3 -> To Workspace5/1  "<xdot>"
  Bus Selector2/4 -> To Workspace12/1  "<NED_wind>"
  Bus Selector2/5 -> To Workspace7/1  "<y_mkplt>"
  Bus Selector2/6 -> To Workspace1/1  "<u_cmd>"
  output_bus/1 -> Bus Selector2/1
  Bus Selector2/7 -> To Workspace3/1  "<u_ulim>"
  Bus Selector2/8 -> To Workspace2/1  "<u_llim>"

== system mach_lib/velocity based angular rate limit ==
  limit_in : Inport
  az_lim : Inport  Port=2
  uvw : Inport  Port=3
  Assignment : Assignment  Elements=q_idx  OutputInitialize=Initialize using input (U1)
  Divide : Product  Inputs=*/  OutScaling=2^-10
  Divide1 : Product  Inputs=*/  OutScaling=2^-10
  Gain : Gain  Gain=-1
  limit1 : MinMax  Function=max  Inputs=2  OutScaling=2^-10  ZeroCross=off
  q_limit : Selector  InputType=Matrix  Elements=2  Rows=-1  Columns=q_idx  InputPortWidth=3
  u : Selector  InputPortWidth=3
  limit_out : Outport
  wires:
  limit_in/1 -> q_limit/1, Assignment/1
  az_lim/1 -> Gain/1
  limit1/1 -> Divide/2
  Divide1/1 -> limit1/1
  Divide/1 -> Assignment/2
  u/1 -> limit1/2
  q_limit/1 -> Divide1/2
  Assignment/1 -> limit_out/1
  uvw/1 -> u/1
  Gain/1 -> Divide/1, Divide1/1

== system mach_lib/wght_cv_diag ==
  rhs : Inport
  Bmat : Inport  Port=2
  wght_cv : Inport  Port=3
  rhs_smn : Outport
  Bmat_smn : Outport  Port=2
  wght_cv_smn : Outport  Port=3
  wires:
  Bmat/1 -> Bmat_smn/1
  rhs/1 -> rhs_smn/1
  wght_cv/1 -> wght_cv_smn/1

== system mach_lib/wght_cv_full ==
  rhs : Inport
  Bmat : Inport  Port=2
  wght_cv : Inport  Port=3
  Constant : Constant  Value=ones(1,num_cv)
  Product1 : Product  Multiplication=Matrix(*)  SaturateOnIntegerOverflow=on  InputSameDT=on
  Product2 : Product  Multiplication=Matrix(*)  SaturateOnIntegerOverflow=on  InputSameDT=on
  rhs_smn : Outport
  Bmat_smn : Outport  Port=2
  wght_cv_smn : Outport  Port=3
  wires:
  Product2/1 -> Bmat_smn/1
  Product1/1 -> rhs_smn/1
  Constant/1 -> wght_cv_smn/1
  wght_cv/1 -> Product2/1, Product1/1
  Bmat/1 -> Product2/2
  rhs/1 -> Product1/2

== system mach_lib/CLAW workspace output/bb debug output ==
  bb_debug : Inport
  Bus Creator : BusCreator  Inputs=13
  Bus Selector6 : BusSelector  OutputSignals=att,att_old,rate,outside,accel,utQu,use_bb,timer,cvd_des,cvd_des_lin
  Bus Selector8 : BusSelector  OutputSignals=dir
  Demux : Demux  Outputs=[1 1 1 1 1 1 3 3 3 3 1 1 3]
  To Workspace35 : ToWorkspace  VariableName=pp_rate  SampleTime=-1  SaveFormat=Array
  To Workspace36 : ToWorkspace  VariableName=pp_att  SampleTime=-1  SaveFormat=Array
  To Workspace37 : ToWorkspace  VariableName=use_bb  SampleTime=-1  SaveFormat=Array
  To Workspace38 : ToWorkspace  VariableName=blend_bb_claw  SampleTime=-1  SaveFormat=Array
  To Workspace39 : ToWorkspace  VariableName=blend_lin_claw  SampleTime=-1  SaveFormat=Array
  To Workspace40 : ToWorkspace  VariableName=pp_utQu  SampleTime=-1  SaveFormat=Array
  To Workspace41 : ToWorkspace  VariableName=outside  SampleTime=-1  SaveFormat=Array
  To Workspace42 : ToWorkspace  VariableName=pp_accel  SampleTime=-1  SaveFormat=Array
  To Workspace43 : ToWorkspace  VariableName=cvd_des_lin  SampleTime=-1  SaveFormat=Array
  bangbang scope : Scope  NumInputPorts=10
      settings: YMin=-2.5~-2.5~0~0~-0.03~0~0~0~-0.9~-1  YMax=0~0~0.125~2000~0.03~2~1~5~0.3~7  SaveName=ScopeData3
  dir scope : Scope
      settings: YMin=-1  YMax=1  SaveName=ScopeData4
  wires:
  bb_debug/1 -> Demux/1
  Bus Selector8/1 -> dir scope/1  "<dir>"
  Bus Selector6/10 -> bangbang scope/10  "<cvd_des_lin>"
  Bus Selector6/9 -> bangbang scope/9  "<cvd_des>"
  Bus Selector6/8 -> bangbang scope/8  "<timer>"
  Bus Selector6/7 -> bangbang scope/7  "<use_bb>"
  Bus Selector6/6 -> bangbang scope/6  "<utQu>"
  Bus Selector6/5 -> bangbang scope/5  "<accel>"
  Bus Selector6/4 -> bangbang scope/4  "<outside>"
  Bus Selector6/3 -> bangbang scope/3  "<rate>"
  Bus Selector6/2 -> bangbang scope/2  "<att_old>"
  Bus Selector6/1 -> bangbang scope/1  "<att>"
  Bus Creator/1 -> Bus Selector8/1, Bus Selector6/1
  Demux/13 -> To Workspace43/1, Bus Creator/13  "cvd_des_lin"
  Demux/12 -> Bus Creator/12  "timer"
  Demux/11 -> To Workspace37/1, Bus Creator/11  "use_bb"
  Demux/10 -> Bus Creator/10  "dir"
  Demux/9 -> Bus Creator/9  "cvd_des"
  Demux/8 -> Bus Creator/8, To Workspace39/1  "blend_lin_claw"
  Demux/7 -> Bus Creator/7, To Workspace38/1  "blend_bb_claw"
  Demux/6 -> Bus Creator/6, To Workspace40/1  "utQu"
  Demux/5 -> Bus Creator/5, To Workspace42/1  "accel"
  Demux/4 -> Bus Creator/4, To Workspace41/1  "outside"
  Demux/2 -> Bus Creator/2  "att_old"
  Demux/3 -> Bus Creator/3, To Workspace35/1  "rate"
  Demux/1 -> Bus Creator/1, To Workspace36/1  "att"

== system mach_lib/P+I+AW+TRIM Control/variable gain comp ==
  int : Inport
  cv : Inport  Port=2
  cvc : Inport  Port=3
  kc : Inport  Port=4
  kb : Inport  Port=5
  ki : Inport  Port=6
  Compare To Zero : simulink/Logic and Bit Operations/Compare To Zero  relop=>  LogicOutDataTypeMode=boolean  ZeroCross=off
  Compare To Zero1 : simulink/Logic and Bit Operations/Compare To Zero  relop===  LogicOutDataTypeMode=boolean  ZeroCross=off
  Demux : Demux  Outputs=2
  Gain : Gain  Gain=1/MACH.dt
  Mux : Mux  Inputs=2
  Mux1 : Mux  Inputs=2
  Product1 : Product  Inputs=*/  RndMeth=Zero
  Product2 : Product  Inputs=3  RndMeth=Zero
  Product3 : Product  Inputs=3  RndMeth=Zero
  Product5 : Product  RndMeth=Zero
  Sum : Sum  Inputs=|++
  Sum1 : Sum  Inputs=|+-
  Sum2 : Sum  Inputs=|-+
  Sum6 : Sum  Inputs=-+|
  Unit Delay : UnitDelay  SampleTime=-1
  int_incr : Outport
  wires:
  cvc/1 -> Mux1/1
  Mux/1 -> Sum6/1, Unit Delay/1
  int/1 -> Sum2/2, Product3/2
  Sum2/1 -> Mux1/2
  cv/1 -> Sum2/1
  Compare To Zero/1 -> Product2/3
  Sum/1 -> Product1/1
  kb/1 -> Product1/2, Mux/2, Product3/1, Product5/2
  kc/1 -> Product5/1
  Product5/1 -> Mux/1
  Sum6/1 -> Product2/2
  Unit Delay/1 -> Compare To Zero/1, Sum6/2
  Mux1/1 -> Product2/1
  Product2/1 -> Demux/1
  Demux/1 -> Sum/1
  Demux/2 -> Sum/2
  Sum1/1 -> int_incr/1
  ki/1 -> Compare To Zero1/1
  Compare To Zero1/1 -> Product3/3
  Product3/1 -> Sum1/2
  Product1/1 -> Gain/1
  Gain/1 -> Sum1/1

== system mach_lib/Stop Sim on Crash/get specific energy ==
  h : Inport
  NEh_dot : Inport  Port=2
  Constant : Constant  Value=constants.g
  Dot Product : simulink/Math Operations/Dot Product  InputSameDT=on  OutDataType=sfix(16)  OutScaling=2^-10  DoSatur=off
  Gain : Gain  Gain=0.5
  Product : Product  RndMeth=Zero
  Sum : Sum  Inputs=|++
  energy : Outport
  wires:
  NEh_dot/1 -> Dot Product/1, Dot Product/2
  Dot Product/1 -> Gain/1
  Gain/1 -> Sum/2
  Sum/1 -> energy/1
  h/1 -> Product/2
  Constant/1 -> Product/1
  Product/1 -> Sum/1

== system mach_lib/claw_main/att_loops ==
  signal_bus : Inport
  outer_cmd : Inport  Port=2
  inner_cmd : Inport  Port=3
  Bus Creator : BusCreator  Inputs=7
  Bus Selector : BusSelector  OutputSignals=control_params.limit_pqr_cmd,x_est.uvw,x_est.e
  Bus Selector4 : BusSelector  OutputSignals=feed_forward.att_ff,mode_sw.int_reset_sw,control_params.att_desdyn
  Demux1 : Demux  Outputs=[ MACH.att_num_u MACH.num_u_throt ]
  Mux2 : Mux  Inputs=2
  P+I+AW+TRIM Control : Subsystem
  compute trim : Subsystem
  dc2mba : utility_lib/dc2mba
  dc2tiltcam : utility_lib/dc2tiltcam
  dc2ypr : utility_lib/dc2ypr
  dyn inv : Subsystem
  e2dc : utility_lib/e2dc
  low pass filter : Subsystem
  select att cmd : Subsystem
  d_cmd : Outport
  outputs : Outport  Port=2
  cmd : Outport  Port=3
  wires:
  Bus Selector4/1 -> low pass filter/3(att_ff)  "<att_ff>"
  low pass filter/2(cvd ff) -> P+I+AW+TRIM Control/3(cvd ff)
  low pass filter/1(cv cmd) -> [cvc], P+I+AW+TRIM Control/2(cv cmd)
  select att cmd/1(e_cmd) -> low pass filter/1(e_cmd)
  [throt_inner] -> select att cmd/2(throt_current)
  Bus Selector/1 -> dyn inv/1(limit_pqr_cmd)  "<limit_pqr_cmd>"
  Bus Selector4/2 -> P+I+AW+TRIM Control/6(reset)  "<int_reset_sw>"
  dyn inv/2(pqr) -> compute trim/3(cmd), Mux2/1
  select att cmd/3(cmd) -> cmd/1
  Bus Selector4/3 -> P+I+AW+TRIM Control/7(x0)  "<att_desdyn>"
  Bus Selector/2 -> dyn inv/2(uvw)  "<uvw>"
  dc2mba/1 -> Bus Creator/7  "mab_cmds"
  dc2ypr/1 -> Bus Creator/6  "rpy_cmds"
  e2dc/1 -> dc2mba/1, dc2ypr/1, dc2tiltcam/1
  [cv] -> Bus Creator/4  "cv"
  dc2tiltcam/1 -> Bus Creator/5  "tiltcam_cmds"
  Demux1/2 -> [throt_inner]
  Demux1/1 -> compute trim/1(inner cmd)
  inner_cmd/1 -> Demux1/1
  Bus Creator/1 -> outputs/1
  [cvc] -> e2dc/1, Bus Creator/3  "cvc"
  select att cmd/2(throt_cmd) -> [throt]
  compute trim/1(trim) -> [trim]
  signal_bus/1 -> low pass filter/2(signal_bus), Bus Selector4/1, select att cmd/4(signal_bus), Bus Selector/1
  [trim] -> P+I+AW+TRIM Control/5(trim)
  dyn inv/1(Bmat) -> compute trim/2(Bmat)
  [cvdex] -> P+I+AW+TRIM Control/4(cvdot extra)
  P+I+AW+TRIM Control/1(cvdot des) -> dyn inv/4(e dot des)
  outer_cmd/1 -> select att cmd/3(outer cmd)
  Bus Selector/3 -> P+I+AW+TRIM Control/1(cv), [cv], dyn inv/3(e nom), select att cmd/1(e_current)  "<e>"
  dyn inv/3(cvdex) -> Bus Creator/1, [cvdex]  "cvdex"
  P+I+AW+TRIM Control/2(int state) -> Bus Creator/2  "integ"
  [throt] -> Mux2/2
  Mux2/1 -> d_cmd/1

== system mach_lib/claw_main/grab ExportedGlobal ==
  debug_output : Inport
  Terminator{1..4,6} (5 alike) : Terminator
  grab cv variables : Subsystem
  grab cvcmd variables : Subsystem
  grab cvdex variables : Subsystem
  grab integrator variables : Subsystem
  grab w_est variables : Subsystem
  wires:
  grab w_est variables/1(Out1) -> Terminator6/1
  grab cv variables/1(Out1) -> Terminator4/1
  grab cvcmd variables/1(Out1) -> Terminator3/1
  grab integrator variables/1(Out1) -> Terminator2/1
  grab cvdex variables/1(Out1) -> Terminator1/1
  debug_output/1 -> grab cvdex variables/1(In1), grab integrator variables/1(In1), grab cvcmd variables/1(In1), grab w_est variables/1(In1), grab cv variables/1(In1)

== system mach_lib/claw_main/input processing ==
  signal_bus : Inport
  scoped_bus : Inport  Port=2
  control_input : Inport  Port=3
  Bus Selector2 : BusSelector  OutputSignals=full_surf
  Bus Selector3 : BusSelector  OutputSignals=engines,mode_sw,command
  Bus Selector4 : BusSelector  OutputSignals=u_old,y_meas.u_meas
  mode dependent stick processing : Subsystem
  modify limits and apply to direct commands : Subsystem
  select att_type : Subsystem
  set control parameters : Subsystem
  cmd_bus : Outport
  control_params : Outport  Port=2
  full_surf : Outport  Port=3
  feed_forward : Outport  Port=4
  engines : Outport  Port=5
  mode_sw : Outport  Port=6
  wires:
  Bus Selector4/2 -> modify limits and apply to direct commands/2(u_meas)  "<u_meas>"
  select att_type/1(mode_sw) -> mode_sw/1
  scoped_bus/1 -> select att_type/1(scoped_bus)
  Bus Selector3/2 -> select att_type/2(mode_sw_in)  "<mode_sw>"
  mode dependent stick processing/2(feed_forward) -> feed_forward/1
  signal_bus/1 -> select att_type/3(signal_bus), mode dependent stick processing/2(signal_bus), Bus Selector4/1, set control parameters/1(signal_bus)
  control_input/1 -> Bus Selector2/1, Bus Selector3/1
  modify limits and apply to direct commands/1(full_surf) -> set control parameters/2(full_surf), full_surf/1
  Bus Selector2/1 -> modify limits and apply to direct commands/3(full_surf_in)  "<full_surf>"
  Bus Selector4/1 -> modify limits and apply to direct commands/1(u_old)  "<u_old>"
  set control parameters/1(control_params) -> control_params/1
  Bus Selector3/3 -> mode dependent stick processing/1(command)  "<command>"
  mode dependent stick processing/1(cmd_bus) -> cmd_bus/1
  Bus Selector3/1 -> engines/1  "<engines>"
